simulink model "BridgeCrossing"  (R2020a)
settings: Solver=FixedStepAuto  StartTime=0.0  StopTime=10.0  FixedStep=1  RelTol=1e-3
libraries: sldvlib x1
settings Model: Creator=jatin  LastModifiedBy=jatin
settings ConfigComp: DVMode=PropertyProving  DVTestSuiteOptimization=Auto  DVDetectOutOfBounds=on

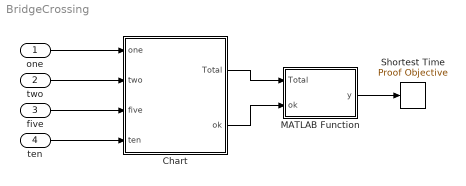
== system BridgeCrossing ==
  one : Inport
  two : Inport  Port=2
  five : Inport  Port=3
  ten : Inport  Port=4
  Chart : Stateflow chart  TreatAsAtomicUnit=on
      settings: PortSchema="{\"entries\":[{\"content\":{\"sides\":[{\"content\":{\"connectorIds\":[\"In1\",\"In2\",\"In3\",\"In4\"]},\"type\":\"ConnectorPlacement.EquallySpacedRectSide\",\"uuid\":\"3d10509f-1c59-4787-b4fe-72fbca6353c5\"},{\"content\":{\"connectorIds\":[\"Out2\",\"Out1\"],\"side\":\"RIGHT\"},\"type\":\"ConnectorPlacement.EquallySpacedRectSide\",\"uuid\":\"d538d11a-30ce-4dac-8c47-4de1dbc60811\"},{\"content\":{\"connectorIds\":[],\"side\":\"TOP\"},\"type\":\"ConnectorPlacement.EquallySpacedRectSide\",\"uuid\":\"623f62af-26ca-45d9-aa13-b0256dfdd7bc\"}]},\"type\":\"ConnectorPlacement.EquallySpacedConnector\",\"uuid\":\"a5432ef1-b18d-4f0e-8ae6-29e7e2427f06\"}],\"packageUris\":[\"http://schema.mathworks.com/mf0/Connector/19700101\"],\"version\":\"1.0\"}"
  MATLAB Function : MATLAB Function  TreatAsAtomicUnit=on
  Shortest Time : sldvlib/Objectives and Constraints/Proof Objective  enabled=on  customAVTBlockType=Proof Objective  intervals=true  dispValues=on  outEnabled=off  enableStopSim=off
      settings: AttributesFormatString=%<intervals>  SourceProductBaseCode=SL
  wires:
  one/1 -> Chart/1(one)
  two/1 -> Chart/2(two)
  five/1 -> Chart/3(five)
  ten/1 -> Chart/4(ten)
  Chart/2(Total) -> MATLAB Function/1(Total)
  Chart/1(ok) -> MATLAB Function/2(ok)
  MATLAB Function/1(y) -> Shortest Time/1

== matlab function BridgeCrossing/MATLAB Function ==
  data: Total input; y output; ok input
function y = fcn(Total,ok)
if Total<18 && ok==0
    y=0;
else
    y=1;
end

== stateflow chart BridgeCrossing/Chart ==
  state Init
  state GOAL
  (default) -> Init : {ok=1;torch=0;one_pos=0;two_pos=0;five_pos=0;ten_pos=0;Total=0;}
  Init -> (junction 14) : {runn();}
  (junction 14) -> (junction 3) [order 1] : [one && one_pos==torch]{one_pos=!one_pos;min=1}
  (junction 14) -> (junction 3) [order 2]
  (junction 6) -> Init [order 2] : {torch=!torch;Total=Total+min}
  (junction 3) -> (junction 4) [order 1] : [two && two_pos==torch]{two_pos=!two_pos;min=2}
  (junction 3) -> (junction 4) [order 2]
  (junction 4) -> (junction 5) [order 2]
  (junction 4) -> (junction 5) [order 1] : [five && five_pos==torch]{five_pos=!five_pos;min=5}
  (junction 5) -> (junction 6) [order 2]
  (junction 5) -> (junction 6) [order 1] : [ten && ten_pos==torch]{ten_pos=!ten_pos;min=10}
  (junction 6) -> GOAL [order 1] : [one_pos && two_pos && five_pos && ten_pos]{ok=0;Total=Total+min}
  data: one input boolean; two input boolean; five input boolean; ten input boolean; ok output boolean; Total output double; five_pos local boolean; min local double; one_pos local boolean; ten_pos local boolean; torch local boolean; two_pos local boolean
  function runn:
    | function runn
    |  sldv.assume(one + two + five + ten <=2);
    |  sldv.assume(one + two + five + ten >0);
    |  sldv.assume((one && one_pos==torch) || (two && two_pos==torch) || (five && five_pos==torch) || (ten && ten_pos==torch));
    | end
